simulink model "validazione_usbl"  (R2020a)
settings: Solver=VariableStepAuto  StartTime=0.0  StopTime=10  RelTol=1e-3
libraries: simulink x1
settings Model: Creator=chiara-s  LastModifiedBy=Rachele
settings DataIOCC: ReturnWorkspaceOutputs=off
settings DebuggingCC: ArithmeticOperatorsInVariantConditions=warning
settings SFSimCC: CustomCodeUndefinedFunction=UseInterfaceOnly

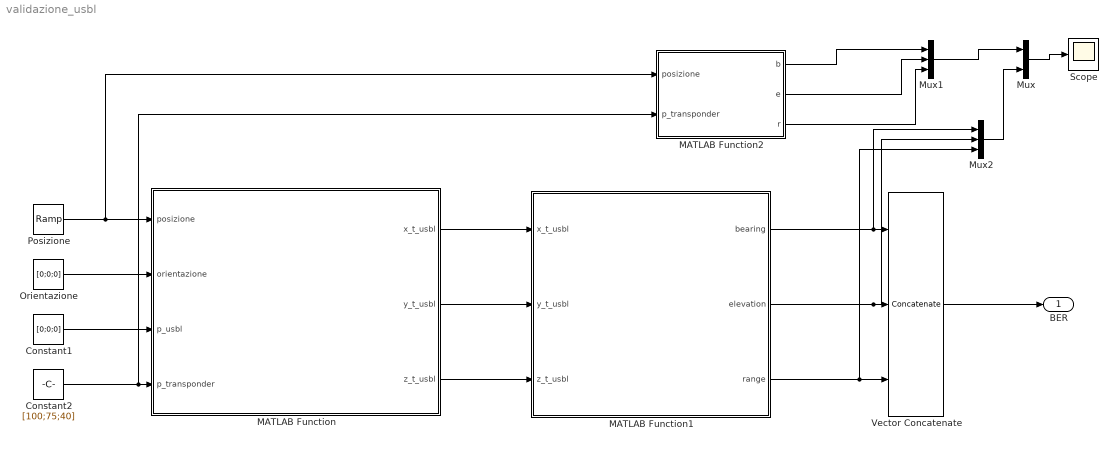
== system validazione_usbl ==
  Constant1 : Constant  Value=[0;0;0]  VectorParams1D=off
  Constant2 : Constant  Value=[100;75;40]  VectorParams1D=off
  MATLAB Function : MATLAB Function  TreatAsAtomicUnit=on
  MATLAB Function1 : MATLAB Function  TreatAsAtomicUnit=on
  MATLAB Function2 : MATLAB Function  TreatAsAtomicUnit=on
  Mux : Mux  Inputs=2
  Mux1 : Mux  Inputs=3
  Mux2 : Mux  Inputs=3
  "Orientazione " : Constant  Value=[0;0;0]  VectorParams1D=off
  Posizione : simulink/Sources/Ramp  slope=[100/5;75/5;0]  start=0  InitialOutput=[0;0;0]  VectorParams1D=off
  Scope : Scope
  Vector Concatenate : Concatenate  NumInputs=3  Mode=Multidimensional array
  BER : Outport  VectorParamsAs1DForOutWhenUnconnected=off
  wires:
  MATLAB Function1/1(bearing) -> Mux2/1, Vector Concatenate/1
  Constant2/1 -> MATLAB Function2/2(p_transponder), MATLAB Function/4(p_transponder)
  Posizione/1 -> MATLAB Function/1(posizione), MATLAB Function2/1(posizione)
  Vector Concatenate/1 -> BER/1
  MATLAB Function1/2(elevation) -> Mux2/2, Vector Concatenate/2
  "Orientazione "/1 -> MATLAB Function/2(orientazione)
  MATLAB Function1/3(range) -> Vector Concatenate/3, Mux2/3
  Constant1/1 -> MATLAB Function/3(p_usbl)
  MATLAB Function/2(y_t_usbl) -> MATLAB Function1/2(y_t_usbl)
  MATLAB Function/1(x_t_usbl) -> MATLAB Function1/1(x_t_usbl)
  MATLAB Function/3(z_t_usbl) -> MATLAB Function1/3(z_t_usbl)
  Mux/1 -> Scope/1
  MATLAB Function2/1(b) -> Mux1/1
  MATLAB Function2/2(e) -> Mux1/2
  MATLAB Function2/3(r) -> Mux1/3
  Mux2/1 -> Mux/2
  Mux1/1 -> Mux/1

== matlab function validazione_usbl/MATLAB Function2 ==
  data: posizione input; b output; p_transponder input; e output; r output
function [b,e,r] = norma(posizione, p_transponder)

r = sqrt((-posizione(1)+p_transponder(1))^2+(-posizione(2)+p_transponder(2))^2+(-posizione(3)+p_transponder(3))^2);
b = atan2((-posizione(2)+p_transponder(2)),(-posizione(1)+p_transponder(1)));
e = asin((-posizione(3)+p_transponder(3))/r);

end

== matlab function validazione_usbl/MATLAB Function ==
  data: posizione input; x_t_usbl output; orientazione input; p_usbl input; p_transponder input; y_t_usbl output; z_t_usbl output
function [x_t_usbl,y_t_usbl,z_t_usbl]= rot_ned_body(posizione,orientazione, p_usbl, p_transponder)
 
 roll = orientazione(1)
 pitch = orientazione(2)
 yaw = orientazione(3)
 xNorth = posizione(1)
 yEast = posizione(2)
 zDown = posizione(3)

 b2transp_ned = p_transponder-[xNorth;yEast;zDown]; %vettore distanza trasponder - veicolo espresso in ned 
 Rx = [1 0 0; 0 cos(roll) -sin(roll); 0 sin(roll) cos(roll)];
 Ry = [cos(pitch) 0 sin(pitch); 0 1 0; -sin(pitch) 0 cos(pitch)];
 Rz = [cos(yaw) -sin(yaw) 0; sin(yaw) cos(yaw) 0; 0 0 1];
 J1 = Rx'*Ry'*Rz'; %matrice di rotazione da ned a body frame 
 transponder_body = J1*b2transp_ned; %posizione transponder in terna body 
 transponder_usbl = transponder_body - p_usbl;  %posizione trasponder in terna usbl 
 x_t_usbl = transponder_usbl(1);
 y_t_usbl = transponder_usbl(2);
 z_t_usbl = transponder_usbl(3);
end

== matlab function validazione_usbl/MATLAB Function1 ==
  data: x_t_usbl input; bearing output; y_t_usbl input; z_t_usbl input; elevation output; range output
function [bearing,elevation,range] = usbl(x_t_usbl, y_t_usbl, z_t_usbl)
 %coordinate sferiche in uscita dal sensore
 range = sqrt((x_t_usbl)^2+(y_t_usbl)^2+(z_t_usbl^2)); 
 elevation = asin(z_t_usbl/range);
 bearing = atan2(y_t_usbl,x_t_usbl); 

 end
